simulink model "Sistema_Seguimiento_Tipo1_Con_Planta_Tipo_0_Sin_Matrices"  (R2016a)
settings: Solver=VariableStepAuto  StartTime=0.0  StopTime=3  RelTol=1e-3
libraries: simulink x1
settings Model: Creator=Abel  LastModifiedBy=Abel

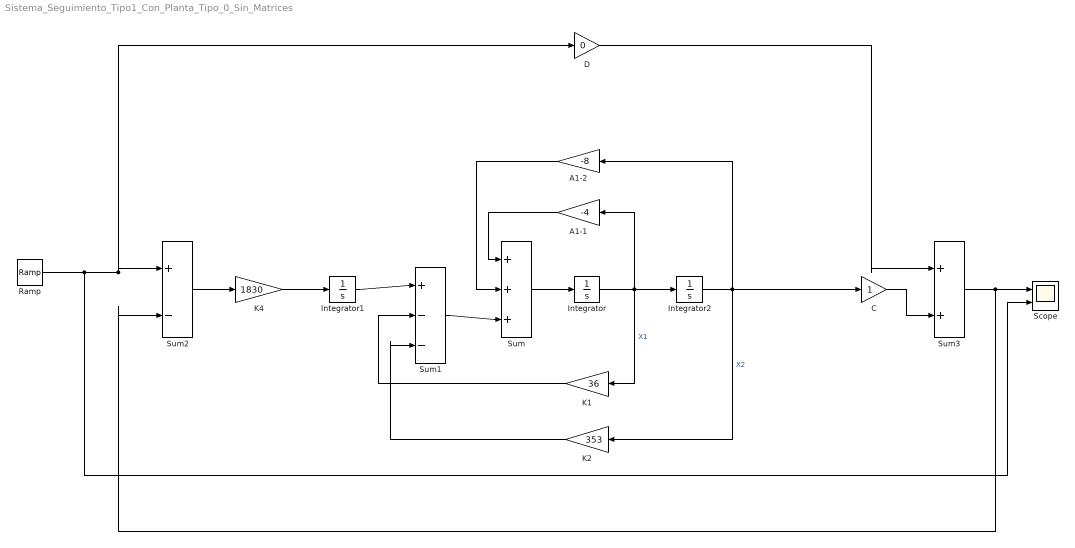
== system Sistema_Seguimiento_Tipo1_Con_Planta_Tipo_0_Sin_Matrices ==
  A1-1 : Gain  Gain=-4
  A1-2 : Gain  Gain=-8
  C : Gain
  D : Gain  Gain=0
  Integrator : Integrator
  Integrator1 : Integrator
  Integrator2 : Integrator
  K1 : Gain  Gain=36
  K2 : Gain  Gain=353
  K4 : Gain  Gain=1830
  Ramp : simulink/Sources/Ramp  slope=1  start=0  X0=0
  Scope : Scope  NumInputPorts=2
  Sum : Sum  Inputs=|+|+|+|
  Sum1 : Sum  Inputs=|+|-|-|
  Sum2 : Sum  Inputs=|+|-|
  Sum3 : Sum  Inputs=|+|+|
  wires:
  Integrator/1 -> K1/1, A1-1/1, Integrator2/1  "X1"
  Sum/1 -> Integrator/1
  A1-1/1 -> Sum/1
  A1-2/1 -> Sum/2
  Integrator2/1 -> C/1, K2/1, A1-2/1  "X2"
  K2/1 -> Sum1/3
  Integrator1/1 -> Sum1/1
  K4/1 -> Integrator1/1
  Sum2/1 -> K4/1
  Ramp/1 -> Scope/2, D/1, Sum2/1
  C/1 -> Sum3/2
  D/1 -> Sum3/1
  Sum3/1 -> Sum2/2, Scope/1
  Sum1/1 -> Sum/3
  K1/1 -> Sum1/2
